simulink model "HalfCar_FrFf"  (R2022a)
settings: Solver=VariableStepAuto  StartTime=0.0  StopTime=10.0  RelTol=1e-3
PreLoadFcn:
  | Lf = 0.9;    % front hub displacement from body gravity center (m)
  | Lr = 1.2;    % rear hub displacement from body gravity center (m)
  | m = 1200;   % body mass (kg)
  | I = 2100;  % body moment of inertia about y-axis in (kg m^2)
  | Kf = 28000;  % front suspension stiffness in (N/m)
  | Kr = 21000;  % rear suspension stiffness in (N/m)
  | Cf = 2500;   % front suspension damping in (N sec/m)
  | Cr = 2000;   % rear suspension damping in (N sec/m)
settings Model: Creator=SK  LastModifiedBy=SK

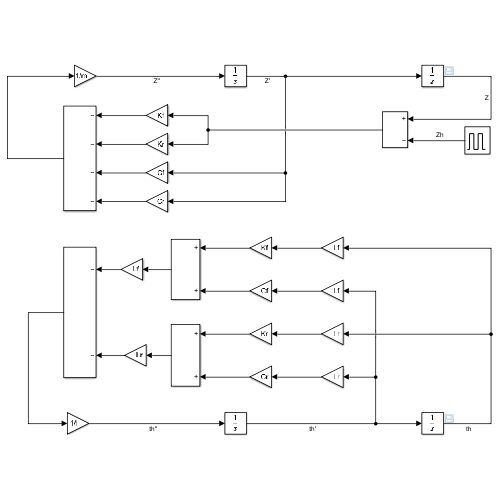
[thumbnail: Simulink's stored preview of the top-level diagram]
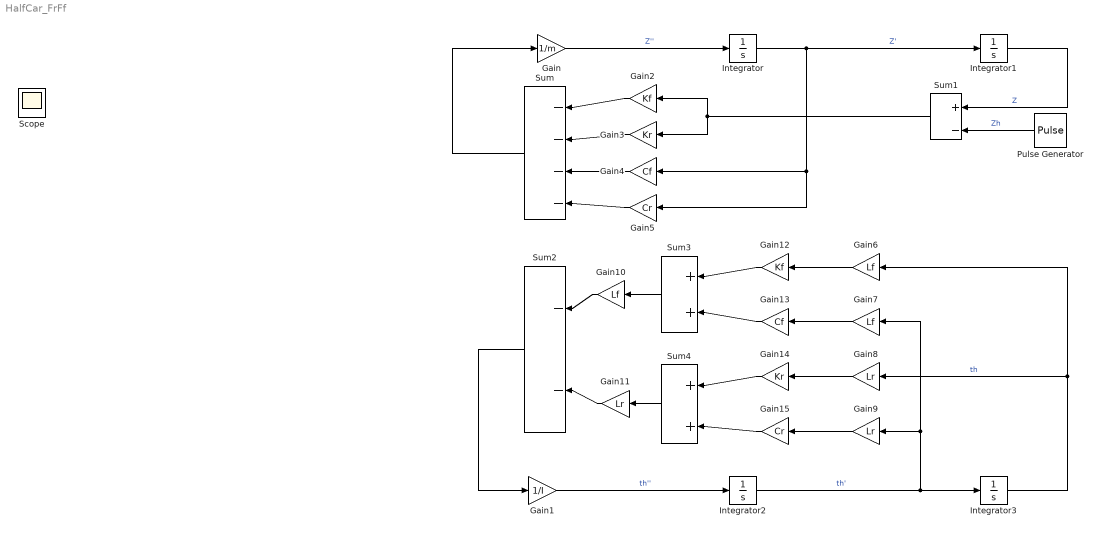
== system HalfCar_FrFf ==
  Gain : Gain  Gain=1/m
  Gain1 : Gain  Gain=1/I
  Gain10 : Gain  Gain=Lf
  Gain11 : Gain  Gain=Lr
  Gain12 : Gain  Gain=Kf
  Gain13 : Gain  Gain=Cf
  Gain14 : Gain  Gain=Kr
  Gain15 : Gain  Gain=Cr
  Gain2 : Gain  Gain=Kf
  Gain3 : Gain  Gain=Kr
  Gain4 : Gain  Gain=Cf
  Gain5 : Gain  Gain=Cr
  Gain6 : Gain  Gain=Lf
  Gain7 : Gain  Gain=Lf
  Gain8 : Gain  Gain=Lr
  Gain9 : Gain  Gain=Lr
  Integrator{,1..3} (4 alike) : Integrator
  Pulse Generator : DiscretePulseGenerator  PulseType=Time based  Period=10  PulseWidth=10  PhaseDelay=2
  Sum : Sum  Inputs=-|-|-|-
  Sum1 : Sum  Inputs=+|-
  Sum2 : Sum  Inputs=-|-
  Sum3 : Sum  Inputs=+|+
  Sum4 : Sum  Inputs=+|+
  Scope : Scope
  wires:
  Integrator/1 -> Gain5/1, Gain4/1, Integrator1/1  "Z'"
  Integrator2/1 -> Gain7/1, Gain9/1, Integrator3/1  "th'"
  Gain/1 -> Integrator/1  "Z''"
  Gain1/1 -> Integrator2/1  "th''"
  Integrator1/1 -> Sum1/1  "Z"
  Integrator3/1 -> Gain6/1, Gain8/1  "th"
  Sum/1 -> Gain/1
  Pulse Generator/1 -> Sum1/2  "Zh"
  Gain5/1 -> Sum/4
  Gain4/1 -> Sum/3
  Gain3/1 -> Sum/2
  Gain2/1 -> Sum/1
  Sum1/1 -> Gain3/1, Gain2/1
  Sum2/1 -> Gain1/1
  Sum4/1 -> Gain11/1
  Sum3/1 -> Gain10/1
  Gain8/1 -> Gain14/1
  Gain10/1 -> Sum2/1
  Gain11/1 -> Sum2/2
  Gain6/1 -> Gain12/1
  Gain12/1 -> Sum3/1
  Gain13/1 -> Sum3/2
  Gain7/1 -> Gain13/1
  Gain14/1 -> Sum4/1
  Gain9/1 -> Gain15/1
  Gain15/1 -> Sum4/2
